simulink model "blank_canvas_ssc_faults"  (R2025b)
settings: Solver=ode1  StartTime=0.0  StopTime=0.1  FixedStep=Ts  RelTol=1e-3  EnableMultiTasking=on
settings Model: Creator=gdudgeon  LastModifiedBy=gdudgeon
settings SolverCC: AlgebraicLoopSolver=TrustRegion  AutoInsertRateTranBlk=on
settings DataIOCC: ExternalInput=[t, load_inputs]  SaveFormat=Array  SaveOutput=off  DSMLogging=off  InspectSignalLogs=on  VisualizeSimOutput=off  SaveTime=off  ReturnWorkspaceOutputs=off
settings OptimizationCC: ExpressionDepthLimit=2147483647.0  LifeSpan=inf
settings DebuggingCC: MergeDetectMultiDrivingBlocksExec=none  SolverPrmCheckMsg=warning  UnconnectedInputMsg=warning  UnconnectedOutputMsg=warning  UnconnectedLineMsg=warning  StateNameClashWarn=warning  SFUnexpectedBacktrackingDiag=warning  SFNoUnconditionalDefaultTransitionDiag=warning  SFExecutionAtInitializationDiag=none  ArithmeticOperatorsInVariantConditions=warning
settings HardwareCC: ProdBitPerPointer=32.0  ProdBitPerSizeT=32.0  ProdBitPerPtrDiffT=32.0  ProdLargestAtomicFloat=None  ProdIntDivRoundTo=Undefined  ProdEndianess=Unspecified  ProdWordSize=32.0  ProdHWDeviceType=32-bit Generic
settings ModelReferenceCC: EnableRefExpFcnMdlSchedulingChecks=on  PropagateSignalLabelsOutOfModel=off
settings SFSimCC: SimUseLocalCustomCode=off  CustomCodeUndefinedFunction=UseInterfaceOnly
settings RTWCC: RTWUseLocalCustomCode=off  GPUComputeCapability=3.5
settings CodeAppCC: StateflowObjectComments=on
settings GRTTargetCC: TargetLangStandard=C89/C90 (ANSI)
settings ConfigComp: CovMetricSettings=dw  CovSaveCumulativeToWorkspaceVar=on  CovSaveSingleToWorkspaceVar=on  CovExternalEMLEnable=off  CovSFcnEnable=off
settings SimscapeCC: SimscapeNormalizeSystem=off
settings ConfigurationSet: Description=SimMechanics 2G

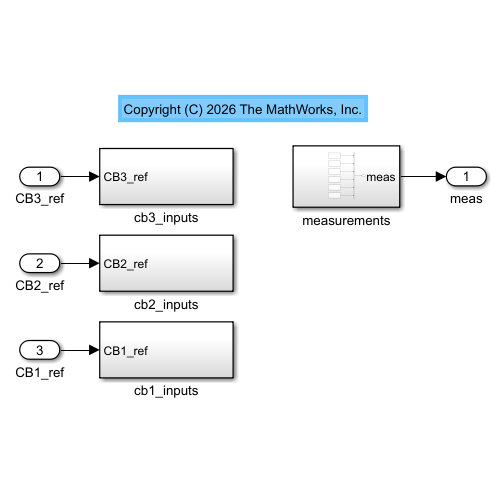
[thumbnail: Simulink's stored preview of the top-level diagram]
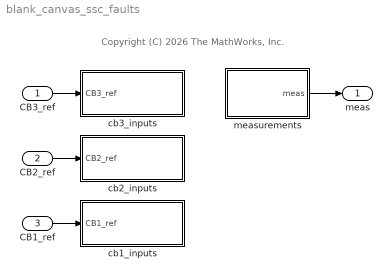
== system blank_canvas_ssc_faults ==
  note: Copyright (C) 2026 The MathWorks, Inc.
  CB3_ref : Inport
  CB2_ref : Inport  Port=2
  CB1_ref : Inport  Port=3
  cb1_inputs : Subsystem
  cb2_inputs : Subsystem
  cb3_inputs : Subsystem
  measurements : Subsystem
  meas : Outport
  wires:
  measurements/1(meas) -> meas/1
  CB3_ref/1 -> cb3_inputs/1(CB3_ref)
  CB2_ref/1 -> cb2_inputs/1(CB2_ref)
  CB1_ref/1 -> cb1_inputs/1(CB1_ref)

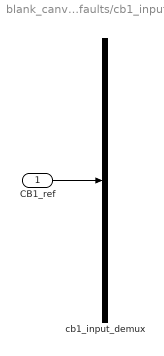
== system blank_canvas_ssc_faults/cb1_inputs ==
  CB1_ref : Inport
  cb1_input_demux : Demux  Outputs=2
  wires:
  CB1_ref/1 -> cb1_input_demux/1

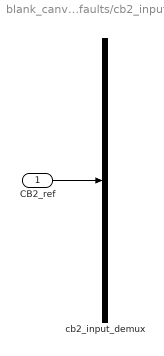
== system blank_canvas_ssc_faults/cb2_inputs ==
  CB2_ref : Inport
  cb2_input_demux : Demux  Outputs=2
  wires:
  CB2_ref/1 -> cb2_input_demux/1

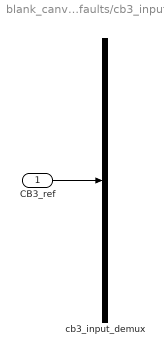
== system blank_canvas_ssc_faults/cb3_inputs ==
  CB3_ref : Inport
  cb3_input_demux : Demux  Outputs=2
  wires:
  CB3_ref/1 -> cb3_input_demux/1

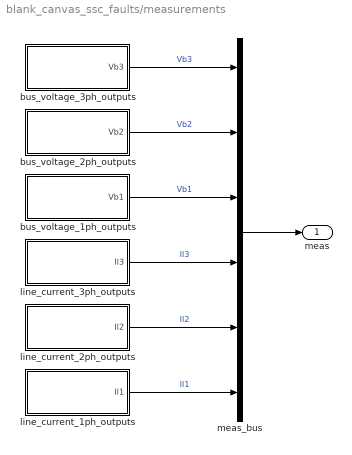
== system blank_canvas_ssc_faults/measurements ==
  bus_voltage_1ph_outputs : Subsystem
  bus_voltage_2ph_outputs : Subsystem
  bus_voltage_3ph_outputs : Subsystem
  line_current_1ph_outputs : Subsystem
  line_current_2ph_outputs : Subsystem
  line_current_3ph_outputs : Subsystem
  meas_bus : BusCreator  Inputs=6
  meas : Outport
  wires:
  bus_voltage_1ph_outputs/1(Vb1) -> meas_bus/3  "Vb1"
  bus_voltage_3ph_outputs/1(Vb3) -> meas_bus/1  "Vb3"
  bus_voltage_2ph_outputs/1(Vb2) -> meas_bus/2  "Vb2"
  meas_bus/1 -> meas/1
  line_current_3ph_outputs/1(Il3) -> meas_bus/4  "Il3"
  line_current_2ph_outputs/1(Il2) -> meas_bus/5  "Il2"
  line_current_1ph_outputs/1(Il1) -> meas_bus/6  "Il1"

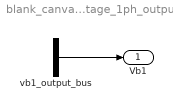
== system blank_canvas_ssc_faults/measurements/bus_voltage_1ph_outputs ==
  vb1_output_bus : BusCreator  Inputs=2
  Vb1 : Outport  VectorParamsAs1DForOutWhenUnconnected=off
  wires:
  vb1_output_bus/1 -> Vb1/1

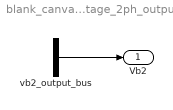
== system blank_canvas_ssc_faults/measurements/bus_voltage_2ph_outputs ==
  vb2_output_bus : BusCreator  Inputs=2
  Vb2 : Outport  VectorParamsAs1DForOutWhenUnconnected=off
  wires:
  vb2_output_bus/1 -> Vb2/1

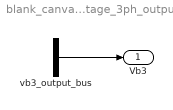
== system blank_canvas_ssc_faults/measurements/bus_voltage_3ph_outputs ==
  vb3_output_bus : BusCreator  Inputs=2
  Vb3 : Outport  VectorParamsAs1DForOutWhenUnconnected=off
  wires:
  vb3_output_bus/1 -> Vb3/1

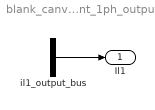
== system blank_canvas_ssc_faults/measurements/line_current_1ph_outputs ==
  il1_output_bus : BusCreator  Inputs=2
  Il1 : Outport  VectorParamsAs1DForOutWhenUnconnected=off
  wires:
  il1_output_bus/1 -> Il1/1

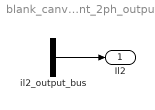
== system blank_canvas_ssc_faults/measurements/line_current_2ph_outputs ==
  il2_output_bus : BusCreator  Inputs=2
  Il2 : Outport  VectorParamsAs1DForOutWhenUnconnected=off
  wires:
  il2_output_bus/1 -> Il2/1

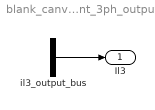
== system blank_canvas_ssc_faults/measurements/line_current_3ph_outputs ==
  il3_output_bus : BusCreator  Inputs=2
  Il3 : Outport  VectorParamsAs1DForOutWhenUnconnected=off
  wires:
  il3_output_bus/1 -> Il3/1
